simulink model "linearizeMdl1"  (R2016b)
settings: Solver=ode23tb  StartTime=0.0  StopTime=10.0  RelTol=1e-3
values from neighbouring files (symbols this model uses):
  x0 = [0.51*pi,0,0.5*pi,0]    [Nonlinearequations.m]    (also in controllerData3.m = [-0.6*pi 0 -0.4*pi 0]; linearizeM.m = [-0.51*pi,0,-0.5*pi,0])
settings Model: Creator=geert  LastModifiedBy=geert

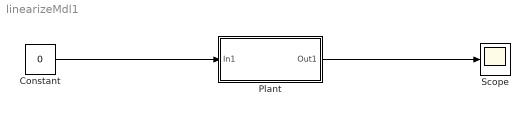
== system linearizeMdl1 ==
  Constant : Constant  Value=0
  Plant : Subsystem
  Scope : Scope
  wires:
  Constant/1 -> Plant/1(In1)
  Plant/1(Out1) -> Scope/1

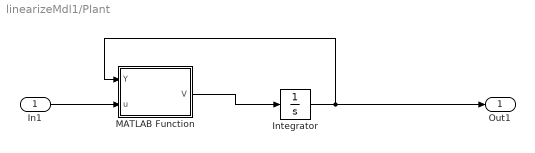
== system linearizeMdl1/Plant ==
  In1 : Inport
  Integrator : Integrator  InitialCondition=x0
  MATLAB Function : MATLAB Function  TreatAsAtomicUnit=on
  Out1 : Outport
  wires:
  Integrator/1 -> MATLAB Function/1(Y), Out1/1
  In1/1 -> MATLAB Function/2(u)
  MATLAB Function/1(V) -> Integrator/1

== matlab function linearizeMdl1/Plant/MATLAB Function ==
  data: Y input; u input; V output
function V = M(Y,u)
%M
%    V = M(Y,U)

%    This function was generated by the Symbolic Math Toolbox version 8.0.
%    09-May-2018 10:56:52

t3 = Y(1);
t4 = Y(3);
t5 = t3-t4;
t2 = cos(t5);
t6 = t2.^2;
t7 = t6.*7.29e-8;
t8 = t7-8.854411999999999e-6;
t9 = 1.0./t8;
t10 = Y(2);
t11 = Y(4);
t12 = cos(t4);
t13 = cos(t3);
t14 = sin(t5);
t15 = t10.^2;
t16 = t3.*2.0;
t17 = t4.*-2.0+t16;
t18 = sin(t17);
t19 = t11.^2;
V = [t10;t9.*t10.*7.649599999999999e-6+t9.*(t13.*1.013074776e-3-t2.*t12.*4.449816e-5)-t2.*t9.*t11.*9.45e-5+t9.*t14.*t19.*1.032696e-5+t9.*t15.*t18.*3.645000000000001e-8+t2.*t9.*u.*4.86e-4;t11;t9.*(t12.*3.8153052e-5-t2.*t13.*7.15149e-6)+t9.*t11.*8.1025e-5-t9.*u.*4.167e-4-t2.*t9.*t10.*5.4e-8-t9.*t14.*t15.*6.2505e-8-t9.*t18.*t19.*3.645000000000001e-8];
